simulink model "LiniowyCalkujace"  (R2015a)
settings: Solver=ode45  StartTime=0.0  StopTime=200  MaxStep=1.5  RelTol=1e-3  AbsTol=1e-6
values from neighbouring files (symbols this model uses):
  a1 = Aw1*sqrt(2*g)    [Dodatkowe.m]    (also in Dodatkowe2.m; ZbiorniczkiLiniowe.m; ZbiorniczkiSumaryczne.m)
  A1 = 3500    [Dodatkowe.m]    (also in Dodatkowe2.m; ZbiorniczkiLiniowe.m; ZbiorniczkiSumaryczne.m)
  A2 = 2000    [Dodatkowe.m]    (also in Dodatkowe2.m; ZbiorniczkiLiniowe.m; ZbiorniczkiSumaryczne.m)
  a2 = Aw2*sqrt(2*g)    [Dodatkowe.m]    (also in Dodatkowe2.m; ZbiorniczkiLiniowe.m; ZbiorniczkiSumaryczne.m)
  df1 = 200    [Dodatkowe.m]    (also in Dodatkowe2.m; ZbiorniczkiLiniowe.m; ZbiorniczkiSumaryczne.m)
  df2 = 0    [Dodatkowe.m]    (also in Dodatkowe2.m; ZbiorniczkiLiniowe.m; ZbiorniczkiSumaryczne.m)
  f1 = wektorf1(i)    [Dodatkowe.m]    (also in Dodatkowe2.m; ZbiorniczkiLiniowe.m; ZbiorniczkiSumaryczne.m)
  f2 = 0    [Dodatkowe.m]    (also in Dodatkowe2.m = 400; ZbiorniczkiLiniowe.m; ZbiorniczkiSumaryczne.m)
  h1 = ((f1.^2)/((Aw1.^2)*2*g))+((f1+f2).^2)/((Aw2.^2)*2*g)    [Dodatkowe.m]    (also in Dodatkowe2.m; ZbiorniczkiLiniowe.m = (f1/a1)+(f1+df2)/a2; ZbiorniczkiSumaryczne.m = (f1/a1)+(f1+df2)/a2)
  h2 = ((f1+f2).^2)/((Aw2.^2)*2*g)    [Dodatkowe.m]    (also in Dodatkowe2.m; ZbiorniczkiLiniowe.m = (f1+df2)/a2; ZbiorniczkiSumaryczne.m = (f1+df2)/a2)
  t1 = 40    [Dodatkowe.m]    (also in Dodatkowe2.m; ZbiorniczkiLiniowe.m; ZbiorniczkiSumaryczne.m)
  t2 = 40    [Dodatkowe.m]    (also in Dodatkowe2.m; ZbiorniczkiLiniowe.m; ZbiorniczkiSumaryczne.m)
settings Model: Creator=LAB320-1552  LastModifiedBy=apuch
settings DebuggingCC: UnderspecifiedInitializationDetection=Classic  MergeDetectMultiDrivingBlocksExec=none  StateNameClashWarn=warning  StrictBusMsg=ErrorOnBusTreatedAsVector

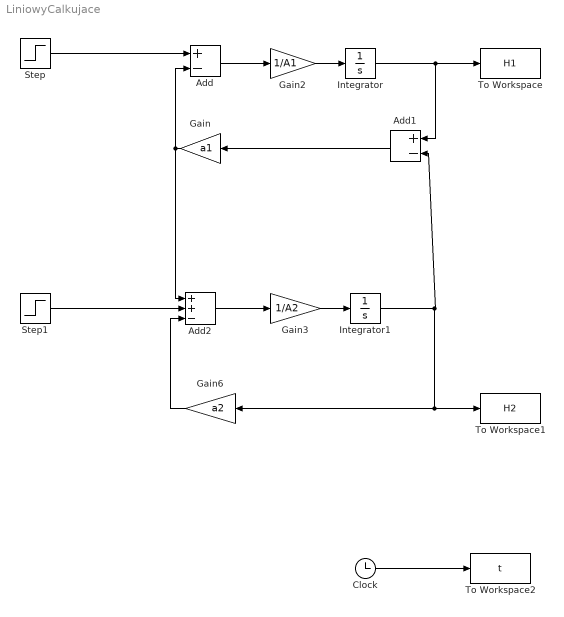
== system LiniowyCalkujace ==
  Add : Sum  Inputs=+-
  Add1 : Sum  Inputs=+-
  Add2 : Sum  Inputs=++-
  Clock : Clock
  Gain : Gain  Gain=a1
  Gain2 : Gain  Gain=1/A1
  Gain3 : Gain  Gain=1/A2
  Gain6 : Gain  Gain=a2
  Integrator : Integrator  InitialCondition=h1
  Integrator1 : Integrator  InitialCondition=h2
  Step : Step  Time=t1  Before=f1  After=f1+df1  SampleTime=0
  Step1 : Step  Time=t2  Before=f2  After=f2+df2  SampleTime=0
  To Workspace : ToWorkspace  VariableName=H1  SampleTime=-1
  To Workspace1 : ToWorkspace  VariableName=H2  SampleTime=-1
  To Workspace2 : ToWorkspace  VariableName=t  SampleTime=-1
  wires:
  Step/1 -> Add/1
  Add/1 -> Gain2/1
  Gain2/1 -> Integrator/1
  Add1/1 -> Gain/1
  Gain/1 -> Add/2, Add2/1
  Integrator/1 -> Add1/1, To Workspace/1
  Step1/1 -> Add2/2
  Add2/1 -> Gain3/1
  Gain3/1 -> Integrator1/1
  Integrator1/1 -> Gain6/1, To Workspace1/1, Add1/2
  Gain6/1 -> Add2/3
  Clock/1 -> To Workspace2/1
